simulink model "TSR_Scenario_005_cs"  (R2014b)
settings: Solver=ode5  SolverMode=SingleTasking  StartTime=0.0  StopTime=inf  FixedStep=1/100  RelTol=1e-3
PreLoadFcn:
  | mbxruntime.callbacks.PreLoadFcn(bdroot);
  | check_NUTS_defined;
  | 
  | assignin('base',['model_closed_' bdroot],false);
  | 
  | addpath('../includes_TSR/includes_TSR');
  | 
  | switch version('-release')
  | case {'2010a', '2010b', '2011a'}
  | addpath('../includes_TSR/ML2010b');
  | otherwise
  | addpath('../includes_TSR/ML2011b');
  | end
PostLoadFcn:
  | mbxruntime.callbacks.PostLoadFcn(bdroot);
InitFcn:
  | mbxruntime.callbacks.InitFcn(bdroot);
StartFcn:
  | mbxruntime.callbacks.StartFcn(bdroot);
StopFcn:
  | mbxruntime.callbacks.StopFcn(bdroot);
model workspace: external: MAT-File .\TSR_Scenario_005_cs_hws.mat (data not in the file)
undefined symbols (not defined in the file or in its folder): InitImageOutputDir, mbxruntime, OrientationPitch, OrientationRoll, PositionX, PositionY, PositionZ, tabledata, warningInitialVelocity, x0
undefined symbols (not defined in the file): SteeringColumn, SteeringWheel, TSR_Scenario_005_cs_00431f954bf6ed0a, TSR_Scenario_005_cs_02a6645fe307ce96, TSR_Scenario_005_cs_0e0d17e780cba748, TSR_Scenario_005_cs_0f94700004e304be, TSR_Scenario_005_cs_13e63084604f23c5, TSR_Scenario_005_cs_18da76569b226b1d, TSR_Scenario_005_cs_19a09eb0dceaf389, TSR_Scenario_005_cs_1d6b1ecf339da803, TSR_Scenario_005_cs_219485daa5a5d171, TSR_Scenario_005_cs_221c03cfb0670d1a, TSR_Scenario_005_cs_22611db63f83df91, TSR_Scenario_005_cs_24324341e1f0fdeb, TSR_Scenario_005_cs_248b5be6aaeb4a32, TSR_Scenario_005_cs_26d69342f02903e6, TSR_Scenario_005_cs_28d4639b4eb6a924, TSR_Scenario_005_cs_2a50646ef6121283, TSR_Scenario_005_cs_2addef8764f78195, TSR_Scenario_005_cs_2c78bb6e92f1c73d, TSR_Scenario_005_cs_330b013c7926b8c0, TSR_Scenario_005_cs_33ac55a3a4bfafc5, TSR_Scenario_005_cs_33d6442482a921b6, TSR_Scenario_005_cs_36fcc85960c1dc31, TSR_Scenario_005_cs_38acb22310967a91, TSR_Scenario_005_cs_3e8855054a9c05f5, TSR_Scenario_005_cs_43d01b44652f0f38, TSR_Scenario_005_cs_43d19ecb630bd754, TSR_Scenario_005_cs_4487c76a87b8c5f1, TSR_Scenario_005_cs_44ceee846c318dfb, TSR_Scenario_005_cs_450a3683cbfdd730, TSR_Scenario_005_cs_464618e49e37493a, TSR_Scenario_005_cs_4880b38df4698ab1, TSR_Scenario_005_cs_4a2b3c7d0abca22e, TSR_Scenario_005_cs_4bd204b8239d5406, TSR_Scenario_005_cs_4de8d67ffbf74a19, TSR_Scenario_005_cs_4f6170ee339e194e, TSR_Scenario_005_cs_50430c8166448bfc, TSR_Scenario_005_cs_53c8f6734eaacbd2, TSR_Scenario_005_cs_543db9a2ff458ebe, TSR_Scenario_005_cs_57976f30ab2edad5, TSR_Scenario_005_cs_5922fccf31372278, TSR_Scenario_005_cs_5a258c940bbe826b, TSR_Scenario_005_cs_6087cc283675db35, TSR_Scenario_005_cs_6246b869963d4acb, TSR_Scenario_005_cs_6352b9f9b72630f9, TSR_Scenario_005_cs_6559b64eceddc3ca, TSR_Scenario_005_cs_6832a8ea8fa66aa4, TSR_Scenario_005_cs_696d53dba69844e5, TSR_Scenario_005_cs_6cabbb37c4ac2dd1, TSR_Scenario_005_cs_6d528aa494c8a952, TSR_Scenario_005_cs_6d945b49f7234fd2, TSR_Scenario_005_cs_6e2ebc771acb2455, TSR_Scenario_005_cs_7897f864ad990cf0, TSR_Scenario_005_cs_7978c65fd141f076, TSR_Scenario_005_cs_7a9ba94120bbe2c7, TSR_Scenario_005_cs_7b108592703c2dc5, TSR_Scenario_005_cs_7cd2f5b09394b811, TSR_Scenario_005_cs_7e1904d085d8f37f, TSR_Scenario_005_cs_7e555208507e0618 ... (+95)
libraries: simulink_extras x59, PreScanSimulinkLibrary x43, simulink x29
(part 12 of 24)

== system TSR_Scenario_005_cs/VISUColorRegion_Shoes_Male_Regular_wSuitcase_1 ==
  VISUColorRegion_Shoes_Male_Regular_wSuitcase_1 : Inport  Tag=inport/ColorRegion  OutDataTypeStr=Bus: PRESCAN_COLOR_DATA  PortDimensions=1  SampleTime=1/100  BusOutputAsStruct=on
  Actuator : S-Function  FunctionName=sfun_ColorActuator  Parameters=mbxruntime.parameters.convert(UniqueID), mbxruntime.parameters.convert(WorldModelSubPath),tabledata, TimeStep  EnableBusSupport=off  mask(PreScan Sink Block: VisuTextureColor){UniqueID=548, WorldModelSubPath=/recolorRegion:name=Shoes/targetColor, TimeStep=1/100}
      mask prompts: UniqueID "Parent Unique Identifier (auto-generated)"; WorldModelSubPath "WM SubPath(auto-generated)"; TimeStep "Simulink time step"
      mask help:
      | The VisuTextureColor block provides a way to adapt the color of a vehicle.
      |
      | For more information, please click Help.
      mask init:
      | [tabledata] = mbxruntime.parameters.table(UniqueID,WorldModelSubPath);
      mask Help: eval('openHelp(230)')
      mask Display: image(imread('TextureColor.png'))
  wires:
  VISUColorRegion_Shoes_Male_Regular_wSuitcase_1/1 -> Actuator/1

== system TSR_Scenario_005_cs/VISUColorRegion_Upper_Body_Female_RegularAni_1 ==
  VISUColorRegion_Upper_Body_Female_RegularAni_1 : Inport  Tag=inport/ColorRegion  OutDataTypeStr=Bus: PRESCAN_COLOR_DATA  PortDimensions=1  SampleTime=1/100  BusOutputAsStruct=on
  Actuator : S-Function  FunctionName=sfun_ColorActuator  Parameters=mbxruntime.parameters.convert(UniqueID), mbxruntime.parameters.convert(WorldModelSubPath),tabledata, TimeStep  EnableBusSupport=off  mask(PreScan Sink Block: VisuTextureColor){UniqueID=592, WorldModelSubPath=/recolorRegion:name=Upper Body/targetColor, TimeStep=1/100}
      mask prompts: UniqueID "Parent Unique Identifier (auto-generated)"; WorldModelSubPath "WM SubPath(auto-generated)"; TimeStep "Simulink time step"
      mask help:
      | The VisuTextureColor block provides a way to adapt the color of a vehicle.
      |
      | For more information, please click Help.
      mask init:
      | [tabledata] = mbxruntime.parameters.table(UniqueID,WorldModelSubPath);
      mask Help: eval('openHelp(230)')
      mask Display: image(imread('TextureColor.png'))
  wires:
  VISUColorRegion_Upper_Body_Female_RegularAni_1/1 -> Actuator/1

== system TSR_Scenario_005_cs/VISUColorRegion_Upper_Body_Female_Regular_wBuggy_1 ==
  VISUColorRegion_Upper_Body_Female_Regular_wBuggy_1 : Inport  Tag=inport/ColorRegion  OutDataTypeStr=Bus: PRESCAN_COLOR_DATA  PortDimensions=1  SampleTime=1/100  BusOutputAsStruct=on
  Actuator : S-Function  FunctionName=sfun_ColorActuator  Parameters=mbxruntime.parameters.convert(UniqueID), mbxruntime.parameters.convert(WorldModelSubPath),tabledata, TimeStep  EnableBusSupport=off  mask(PreScan Sink Block: VisuTextureColor){UniqueID=539, WorldModelSubPath=/recolorRegion:name=Upper Body/targetColor, TimeStep=1/100}
      mask prompts: UniqueID "Parent Unique Identifier (auto-generated)"; WorldModelSubPath "WM SubPath(auto-generated)"; TimeStep "Simulink time step"
      mask help:
      | The VisuTextureColor block provides a way to adapt the color of a vehicle.
      |
      | For more information, please click Help.
      mask init:
      | [tabledata] = mbxruntime.parameters.table(UniqueID,WorldModelSubPath);
      mask Help: eval('openHelp(230)')
      mask Display: image(imread('TextureColor.png'))
  wires:
  VISUColorRegion_Upper_Body_Female_Regular_wBuggy_1/1 -> Actuator/1

== system TSR_Scenario_005_cs/VISUColorRegion_Upper_Body_Male_RegularAni_1 ==
  VISUColorRegion_Upper_Body_Male_RegularAni_1 : Inport  Tag=inport/ColorRegion  OutDataTypeStr=Bus: PRESCAN_COLOR_DATA  PortDimensions=1  SampleTime=1/100  BusOutputAsStruct=on
  Actuator : S-Function  FunctionName=sfun_ColorActuator  Parameters=mbxruntime.parameters.convert(UniqueID), mbxruntime.parameters.convert(WorldModelSubPath),tabledata, TimeStep  EnableBusSupport=off  mask(PreScan Sink Block: VisuTextureColor){UniqueID=316, WorldModelSubPath=/recolorRegion:name=Upper Body/targetColor, TimeStep=1/100}
      mask prompts: UniqueID "Parent Unique Identifier (auto-generated)"; WorldModelSubPath "WM SubPath(auto-generated)"; TimeStep "Simulink time step"
      mask help:
      | The VisuTextureColor block provides a way to adapt the color of a vehicle.
      |
      | For more information, please click Help.
      mask init:
      | [tabledata] = mbxruntime.parameters.table(UniqueID,WorldModelSubPath);
      mask Help: eval('openHelp(230)')
      mask Display: image(imread('TextureColor.png'))
  wires:
  VISUColorRegion_Upper_Body_Male_RegularAni_1/1 -> Actuator/1

== system TSR_Scenario_005_cs/VISUColorRegion_Upper_Body_Male_Regular_wBackpack_1 ==
  VISUColorRegion_Upper_Body_Male_Regular_wBackpack_1 : Inport  Tag=inport/ColorRegion  OutDataTypeStr=Bus: PRESCAN_COLOR_DATA  PortDimensions=1  SampleTime=1/100  BusOutputAsStruct=on
  Actuator : S-Function  FunctionName=sfun_ColorActuator  Parameters=mbxruntime.parameters.convert(UniqueID), mbxruntime.parameters.convert(WorldModelSubPath),tabledata, TimeStep  EnableBusSupport=off  mask(PreScan Sink Block: VisuTextureColor){UniqueID=595, WorldModelSubPath=/recolorRegion:name=Upper Body/targetColor, TimeStep=1/100}
      mask prompts: UniqueID "Parent Unique Identifier (auto-generated)"; WorldModelSubPath "WM SubPath(auto-generated)"; TimeStep "Simulink time step"
      mask help:
      | The VisuTextureColor block provides a way to adapt the color of a vehicle.
      |
      | For more information, please click Help.
      mask init:
      | [tabledata] = mbxruntime.parameters.table(UniqueID,WorldModelSubPath);
      mask Help: eval('openHelp(230)')
      mask Display: image(imread('TextureColor.png'))
  wires:
  VISUColorRegion_Upper_Body_Male_Regular_wBackpack_1/1 -> Actuator/1

== system TSR_Scenario_005_cs/VISUColorRegion_Upper_Body_Male_Regular_wBicycle_1 ==
  VISUColorRegion_Upper_Body_Male_Regular_wBicycle_1 : Inport  Tag=inport/ColorRegion  OutDataTypeStr=Bus: PRESCAN_COLOR_DATA  PortDimensions=1  SampleTime=1/100  BusOutputAsStruct=on
  Actuator : S-Function  FunctionName=sfun_ColorActuator  Parameters=mbxruntime.parameters.convert(UniqueID), mbxruntime.parameters.convert(WorldModelSubPath),tabledata, TimeStep  EnableBusSupport=off  mask(PreScan Sink Block: VisuTextureColor){UniqueID=542, WorldModelSubPath=/recolorRegion:name=Upper Body/targetColor, TimeStep=1/100}
      mask prompts: UniqueID "Parent Unique Identifier (auto-generated)"; WorldModelSubPath "WM SubPath(auto-generated)"; TimeStep "Simulink time step"
      mask help:
      | The VisuTextureColor block provides a way to adapt the color of a vehicle.
      |
      | For more information, please click Help.
      mask init:
      | [tabledata] = mbxruntime.parameters.table(UniqueID,WorldModelSubPath);
      mask Help: eval('openHelp(230)')
      mask Display: image(imread('TextureColor.png'))
  wires:
  VISUColorRegion_Upper_Body_Male_Regular_wBicycle_1/1 -> Actuator/1

== system TSR_Scenario_005_cs/VISUColorRegion_Upper_Body_Male_Regular_wSuitcase_1 ==
  VISUColorRegion_Upper_Body_Male_Regular_wSuitcase_1 : Inport  Tag=inport/ColorRegion  OutDataTypeStr=Bus: PRESCAN_COLOR_DATA  PortDimensions=1  SampleTime=1/100  BusOutputAsStruct=on
  Actuator : S-Function  FunctionName=sfun_ColorActuator  Parameters=mbxruntime.parameters.convert(UniqueID), mbxruntime.parameters.convert(WorldModelSubPath),tabledata, TimeStep  EnableBusSupport=off  mask(PreScan Sink Block: VisuTextureColor){UniqueID=548, WorldModelSubPath=/recolorRegion:name=Upper Body/targetColor, TimeStep=1/100}
      mask prompts: UniqueID "Parent Unique Identifier (auto-generated)"; WorldModelSubPath "WM SubPath(auto-generated)"; TimeStep "Simulink time step"
      mask help:
      | The VisuTextureColor block provides a way to adapt the color of a vehicle.
      |
      | For more information, please click Help.
      mask init:
      | [tabledata] = mbxruntime.parameters.table(UniqueID,WorldModelSubPath);
      mask Help: eval('openHelp(230)')
      mask Display: image(imread('TextureColor.png'))
  wires:
  VISUColorRegion_Upper_Body_Male_Regular_wSuitcase_1/1 -> Actuator/1

== system TSR_Scenario_005_cs/WheelL0_Audi_A8_1 ==
  WheelL0_Audi_A8_1 : Inport  Tag=inport/JointActuator  OutDataTypeStr=Bus: PRESCAN_POSE_DATA  SampleTime=1/100  BusOutputAsStruct=on
  Actuator : Subsystem  Tag=VisuJoint  mask(PreScan Sink Block: VisuJoint){UniqueID=210, Translate_ObjectID3D=Audi_A8_1.WheelL0, Rotate_ObjectID3D=Audi_A8_1.WheelL0, TimeStep=1/100, DisplayName=[]}
      mask prompts: UniqueID "Parent Unique ID"; Translate_ObjectID3D "Translate Object Name"; Rotate_ObjectID3D "Rotate Object Name"; TimeStep "Simulation Step"; DisplayName "Display Name"
      mask help:
      | The VisuJoint block provides a way to adapt the location and orientation of a part of an object.
      |
      | For more information, please click Help.
      settings: DeleteFcn=PreScanBlockDeleteFcn;
      mask Help: eval('openHelp(223)')
      mask Display: image(imread('Joint.png'))
  wires:
  WheelL0_Audi_A8_1/1 -> Actuator/1(Joint)

== system TSR_Scenario_005_cs/WheelL0_Ford_Fiesta_1 ==
  WheelL0_Ford_Fiesta_1 : Inport  Tag=inport/JointActuator  OutDataTypeStr=Bus: PRESCAN_POSE_DATA  SampleTime=1/100  BusOutputAsStruct=on
  Actuator : Subsystem  Tag=VisuJoint  mask(PreScan Sink Block: VisuJoint){UniqueID=231, Translate_ObjectID3D=Ford_Fiesta_1.WheelL0, Rotate_ObjectID3D=Ford_Fiesta_1.WheelL0, TimeStep=1/100, DisplayName=[]}
      mask prompts: UniqueID "Parent Unique ID"; Translate_ObjectID3D "Translate Object Name"; Rotate_ObjectID3D "Rotate Object Name"; TimeStep "Simulation Step"; DisplayName "Display Name"
      mask help:
      | The VisuJoint block provides a way to adapt the location and orientation of a part of an object.
      |
      | For more information, please click Help.
      settings: DeleteFcn=PreScanBlockDeleteFcn;
      mask Help: eval('openHelp(223)')
      mask Display: image(imread('Joint.png'))
  wires:
  WheelL0_Ford_Fiesta_1/1 -> Actuator/1(Joint)

== system TSR_Scenario_005_cs/WheelL0_Toyota_Yaris_1 ==
  WheelL0_Toyota_Yaris_1 : Inport  Tag=inport/JointActuator  OutDataTypeStr=Bus: PRESCAN_POSE_DATA  SampleTime=1/100  BusOutputAsStruct=on
  Actuator : Subsystem  Tag=VisuJoint  mask(PreScan Sink Block: VisuJoint){UniqueID=225, Translate_ObjectID3D=Toyota_Yaris_1.WheelL0, Rotate_ObjectID3D=Toyota_Yaris_1.WheelL0, TimeStep=1/100, DisplayName=[]}
      mask prompts: UniqueID "Parent Unique ID"; Translate_ObjectID3D "Translate Object Name"; Rotate_ObjectID3D "Rotate Object Name"; TimeStep "Simulation Step"; DisplayName "Display Name"
      mask help:
      | The VisuJoint block provides a way to adapt the location and orientation of a part of an object.
      |
      | For more information, please click Help.
      settings: DeleteFcn=PreScanBlockDeleteFcn;
      mask Help: eval('openHelp(223)')
      mask Display: image(imread('Joint.png'))
  wires:
  WheelL0_Toyota_Yaris_1/1 -> Actuator/1(Joint)

== system TSR_Scenario_005_cs/WheelL1_Audi_A8_1 ==
  WheelL1_Audi_A8_1 : Inport  Tag=inport/JointActuator  OutDataTypeStr=Bus: PRESCAN_POSE_DATA  SampleTime=1/100  BusOutputAsStruct=on
  Actuator : Subsystem  Tag=VisuJoint  mask(PreScan Sink Block: VisuJoint){UniqueID=210, Translate_ObjectID3D=Audi_A8_1.WheelL1, Rotate_ObjectID3D=Audi_A8_1.WheelL1, TimeStep=1/100, DisplayName=[]}
      mask prompts: UniqueID "Parent Unique ID"; Translate_ObjectID3D "Translate Object Name"; Rotate_ObjectID3D "Rotate Object Name"; TimeStep "Simulation Step"; DisplayName "Display Name"
      mask help:
      | The VisuJoint block provides a way to adapt the location and orientation of a part of an object.
      |
      | For more information, please click Help.
      settings: DeleteFcn=PreScanBlockDeleteFcn;
      mask Help: eval('openHelp(223)')
      mask Display: image(imread('Joint.png'))
  wires:
  WheelL1_Audi_A8_1/1 -> Actuator/1(Joint)

== system TSR_Scenario_005_cs/WheelL1_Ford_Fiesta_1 ==
  WheelL1_Ford_Fiesta_1 : Inport  Tag=inport/JointActuator  OutDataTypeStr=Bus: PRESCAN_POSE_DATA  SampleTime=1/100  BusOutputAsStruct=on
  Actuator : Subsystem  Tag=VisuJoint  mask(PreScan Sink Block: VisuJoint){UniqueID=231, Translate_ObjectID3D=Ford_Fiesta_1.WheelL1, Rotate_ObjectID3D=Ford_Fiesta_1.WheelL1, TimeStep=1/100, DisplayName=[]}
      mask prompts: UniqueID "Parent Unique ID"; Translate_ObjectID3D "Translate Object Name"; Rotate_ObjectID3D "Rotate Object Name"; TimeStep "Simulation Step"; DisplayName "Display Name"
      mask help:
      | The VisuJoint block provides a way to adapt the location and orientation of a part of an object.
      |
      | For more information, please click Help.
      settings: DeleteFcn=PreScanBlockDeleteFcn;
      mask Help: eval('openHelp(223)')
      mask Display: image(imread('Joint.png'))
  wires:
  WheelL1_Ford_Fiesta_1/1 -> Actuator/1(Joint)

== system TSR_Scenario_005_cs/WheelL1_Toyota_Yaris_1 ==
  WheelL1_Toyota_Yaris_1 : Inport  Tag=inport/JointActuator  OutDataTypeStr=Bus: PRESCAN_POSE_DATA  SampleTime=1/100  BusOutputAsStruct=on
  Actuator : Subsystem  Tag=VisuJoint  mask(PreScan Sink Block: VisuJoint){UniqueID=225, Translate_ObjectID3D=Toyota_Yaris_1.WheelL1, Rotate_ObjectID3D=Toyota_Yaris_1.WheelL1, TimeStep=1/100, DisplayName=[]}
      mask prompts: UniqueID "Parent Unique ID"; Translate_ObjectID3D "Translate Object Name"; Rotate_ObjectID3D "Rotate Object Name"; TimeStep "Simulation Step"; DisplayName "Display Name"
      mask help:
      | The VisuJoint block provides a way to adapt the location and orientation of a part of an object.
      |
      | For more information, please click Help.
      settings: DeleteFcn=PreScanBlockDeleteFcn;
      mask Help: eval('openHelp(223)')
      mask Display: image(imread('Joint.png'))
  wires:
  WheelL1_Toyota_Yaris_1/1 -> Actuator/1(Joint)

== system TSR_Scenario_005_cs/WheelR0_Audi_A8_1 ==
  WheelR0_Audi_A8_1 : Inport  Tag=inport/JointActuator  OutDataTypeStr=Bus: PRESCAN_POSE_DATA  SampleTime=1/100  BusOutputAsStruct=on
  Actuator : Subsystem  Tag=VisuJoint  mask(PreScan Sink Block: VisuJoint){UniqueID=210, Translate_ObjectID3D=Audi_A8_1.WheelR0, Rotate_ObjectID3D=Audi_A8_1.WheelR0, TimeStep=1/100, DisplayName=[]}
      mask prompts: UniqueID "Parent Unique ID"; Translate_ObjectID3D "Translate Object Name"; Rotate_ObjectID3D "Rotate Object Name"; TimeStep "Simulation Step"; DisplayName "Display Name"
      mask help:
      | The VisuJoint block provides a way to adapt the location and orientation of a part of an object.
      |
      | For more information, please click Help.
      settings: DeleteFcn=PreScanBlockDeleteFcn;
      mask Help: eval('openHelp(223)')
      mask Display: image(imread('Joint.png'))
  wires:
  WheelR0_Audi_A8_1/1 -> Actuator/1(Joint)

== system TSR_Scenario_005_cs/WheelR0_Ford_Fiesta_1 ==
  WheelR0_Ford_Fiesta_1 : Inport  Tag=inport/JointActuator  OutDataTypeStr=Bus: PRESCAN_POSE_DATA  SampleTime=1/100  BusOutputAsStruct=on
  Actuator : Subsystem  Tag=VisuJoint  mask(PreScan Sink Block: VisuJoint){UniqueID=231, Translate_ObjectID3D=Ford_Fiesta_1.WheelR0, Rotate_ObjectID3D=Ford_Fiesta_1.WheelR0, TimeStep=1/100, DisplayName=[]}
      mask prompts: UniqueID "Parent Unique ID"; Translate_ObjectID3D "Translate Object Name"; Rotate_ObjectID3D "Rotate Object Name"; TimeStep "Simulation Step"; DisplayName "Display Name"
      mask help:
      | The VisuJoint block provides a way to adapt the location and orientation of a part of an object.
      |
      | For more information, please click Help.
      settings: DeleteFcn=PreScanBlockDeleteFcn;
      mask Help: eval('openHelp(223)')
      mask Display: image(imread('Joint.png'))
  wires:
  WheelR0_Ford_Fiesta_1/1 -> Actuator/1(Joint)

== system TSR_Scenario_005_cs/WheelR0_Toyota_Yaris_1 ==
  WheelR0_Toyota_Yaris_1 : Inport  Tag=inport/JointActuator  OutDataTypeStr=Bus: PRESCAN_POSE_DATA  SampleTime=1/100  BusOutputAsStruct=on
  Actuator : Subsystem  Tag=VisuJoint  mask(PreScan Sink Block: VisuJoint){UniqueID=225, Translate_ObjectID3D=Toyota_Yaris_1.WheelR0, Rotate_ObjectID3D=Toyota_Yaris_1.WheelR0, TimeStep=1/100, DisplayName=[]}
      mask prompts: UniqueID "Parent Unique ID"; Translate_ObjectID3D "Translate Object Name"; Rotate_ObjectID3D "Rotate Object Name"; TimeStep "Simulation Step"; DisplayName "Display Name"
      mask help:
      | The VisuJoint block provides a way to adapt the location and orientation of a part of an object.
      |
      | For more information, please click Help.
      settings: DeleteFcn=PreScanBlockDeleteFcn;
      mask Help: eval('openHelp(223)')
      mask Display: image(imread('Joint.png'))
  wires:
  WheelR0_Toyota_Yaris_1/1 -> Actuator/1(Joint)

== system TSR_Scenario_005_cs/WheelR1_Audi_A8_1 ==
  WheelR1_Audi_A8_1 : Inport  Tag=inport/JointActuator  OutDataTypeStr=Bus: PRESCAN_POSE_DATA  SampleTime=1/100  BusOutputAsStruct=on
  Actuator : Subsystem  Tag=VisuJoint  mask(PreScan Sink Block: VisuJoint){UniqueID=210, Translate_ObjectID3D=Audi_A8_1.WheelR1, Rotate_ObjectID3D=Audi_A8_1.WheelR1, TimeStep=1/100, DisplayName=[]}
      mask prompts: UniqueID "Parent Unique ID"; Translate_ObjectID3D "Translate Object Name"; Rotate_ObjectID3D "Rotate Object Name"; TimeStep "Simulation Step"; DisplayName "Display Name"
      mask help:
      | The VisuJoint block provides a way to adapt the location and orientation of a part of an object.
      |
      | For more information, please click Help.
      settings: DeleteFcn=PreScanBlockDeleteFcn;
      mask Help: eval('openHelp(223)')
      mask Display: image(imread('Joint.png'))
  wires:
  WheelR1_Audi_A8_1/1 -> Actuator/1(Joint)

== system TSR_Scenario_005_cs/WheelR1_Ford_Fiesta_1 ==
  WheelR1_Ford_Fiesta_1 : Inport  Tag=inport/JointActuator  OutDataTypeStr=Bus: PRESCAN_POSE_DATA  SampleTime=1/100  BusOutputAsStruct=on
  Actuator : Subsystem  Tag=VisuJoint  mask(PreScan Sink Block: VisuJoint){UniqueID=231, Translate_ObjectID3D=Ford_Fiesta_1.WheelR1, Rotate_ObjectID3D=Ford_Fiesta_1.WheelR1, TimeStep=1/100, DisplayName=[]}
      mask prompts: UniqueID "Parent Unique ID"; Translate_ObjectID3D "Translate Object Name"; Rotate_ObjectID3D "Rotate Object Name"; TimeStep "Simulation Step"; DisplayName "Display Name"
      mask help:
      | The VisuJoint block provides a way to adapt the location and orientation of a part of an object.
      |
      | For more information, please click Help.
      settings: DeleteFcn=PreScanBlockDeleteFcn;
      mask Help: eval('openHelp(223)')
      mask Display: image(imread('Joint.png'))
  wires:
  WheelR1_Ford_Fiesta_1/1 -> Actuator/1(Joint)

== system TSR_Scenario_005_cs/WheelR1_Toyota_Yaris_1 ==
  WheelR1_Toyota_Yaris_1 : Inport  Tag=inport/JointActuator  OutDataTypeStr=Bus: PRESCAN_POSE_DATA  SampleTime=1/100  BusOutputAsStruct=on
  Actuator : Subsystem  Tag=VisuJoint  mask(PreScan Sink Block: VisuJoint){UniqueID=225, Translate_ObjectID3D=Toyota_Yaris_1.WheelR1, Rotate_ObjectID3D=Toyota_Yaris_1.WheelR1, TimeStep=1/100, DisplayName=[]}
      mask prompts: UniqueID "Parent Unique ID"; Translate_ObjectID3D "Translate Object Name"; Rotate_ObjectID3D "Rotate Object Name"; TimeStep "Simulation Step"; DisplayName "Display Name"
      mask help:
      | The VisuJoint block provides a way to adapt the location and orientation of a part of an object.
      |
      | For more information, please click Help.
      settings: DeleteFcn=PreScanBlockDeleteFcn;
      mask Help: eval('openHelp(223)')
      mask Display: image(imread('Joint.png'))
  wires:
  WheelR1_Toyota_Yaris_1/1 -> Actuator/1(Joint)

== system TSR_Scenario_005_cs/Actros_1860_1/SELF_Demux ==
  SELF : Inport  OutDataTypeStr=Bus: PRESCAN_SELFSENSORDATA
  Bus Selector : BusSelector  OutputSignals=PositionX,PositionY,PositionZ,OrientationRoll,OrientationPitch,OrientationYaw,Velocity,Yaw_rate,Lat,Long,Alt
  Demux2 : Demux  Outputs=3
  Gain : Gain  Gain=180/pi
  Gain1 : Gain  Gain=180/pi
  Vector Concatenate1 : Concatenate  NumInputs=3
  compas converter : Subsystem
  x [m] : Outport
  y [m] : Outport  Port=2
  z [m] : Outport  Port=3
  rotx [deg] : Outport  Port=4
  roty [deg] : Outport  Port=5
  rotz [deg] : Outport  Port=6
  GPS lat [deg] : Outport  Port=7
  GPS long [deg] : Outport  Port=8
  GPS alt [m] : Outport  Port=9
  velocity [m/s] : Outport  Port=10
  heading [deg] : Outport  Port=11
  yaw rate [deg/s] : Outport  Port=12
  wires:
  Bus Selector/11 -> GPS alt [m]/1  "<Alt>"
  Bus Selector/10 -> GPS long [deg]/1  "<Long>"
  Bus Selector/9 -> GPS lat [deg]/1  "<Lat>"
  Bus Selector/8 -> Gain1/1  "<Yaw_rate>"
  Bus Selector/7 -> velocity [m/s]/1  "<Velocity>"
  Bus Selector/6 -> compas converter/1(rotz [rad]), Vector Concatenate1/3  "<OrientationYaw>"
  Bus Selector/5 -> Vector Concatenate1/2  "<OrientationPitch>"
  Bus Selector/4 -> Vector Concatenate1/1  "<OrientationRoll>"
  Vector Concatenate1/1 -> Gain/1
  Bus Selector/3 -> z [m]/1  "<PositionZ>"
  Bus Selector/2 -> y [m]/1  "<PositionY>"
  Bus Selector/1 -> x [m]/1  "<PositionX>"
  SELF/1 -> Bus Selector/1
  Gain/1 -> Demux2/1
  Demux2/1 -> rotx [deg]/1
  Demux2/2 -> roty [deg]/1
  Demux2/3 -> rotz [deg]/1
  compas converter/1(heading [deg]) -> heading [deg]/1
  Gain1/1 -> yaw rate [deg/s]/1

== system TSR_Scenario_005_cs/Actros_2541_1/Dynamics_Empty ==
  note: For state mode 'Dynamic' positions
      | are not taken into account, as they
      | are computed by integrating velocity.
      | Click annotation for Help.
  Ground_{1..9} (9 alike) : Ground
  MuxState : Subsystem  Tag=mux/State  mask(Empty Dynamics State Block){positioningmode=on, TimeStep=1/100}
      mask prompts: positioningmode "Positioning Mode"; TimeStep "Auto Assigned: Time Step [s]"
      mask help:
      | Build the state of an actor based on user input.
      | The user can either use positioning mode or dynamics mode.
      | - When using positioning mode the position and orientation of the actor are set directly based on the input. Expected input is relative to the initial position and orientation of the actor. It's also possible to specify the velocity of the actor, though this input isn't used, only passed on.
      | - When using dynamics mode the position input is ignored. Expected input is velocity and orientation. The velocity is relative the current orientation of the actor, while orientation is relative to its initial orientation. The position of the actor is calculated based on the velocity and orientation given.
      settings: DeleteFcn=PreScanBlockDeleteFcn;
  STATE_Actros_2541_1 : Subsystem  Tag=mux/StatePort  Priority=0  LoadFcn=load PrescanStateActuatorData  mask(PreScan Sink Block: State){x0=TSR_Scenario_005_cs_81f8b291f80d3bb5, y0=TSR_Scenario_005_cs_b36b553bfda2753f, z0=TSR_Scenario_005_cs_ceb708ef07534e98, Roll0=TSR_Scenario_005_cs_7e1904d085d8f37f, Pitch0=TSR_Scenario_005_cs_cf6308a405ae1ed0, Yaw0=TSR_Scenario_005_cs_3e8855054a9c05f5, TimeStep=1/100}
      mask prompts: x0 "Ini x-position VEHICLE wrt GLOBAL axis system [m]"; y0 "Ini y-position VEHICLE wrt GLOBAL axis system [m]"; z0 "Ini z-position VEHICLE wrt GLOBAL axis system [m]"; Roll0 "Ini roll-angle BODY wrt VEHICLE axis system [deg]"; Pitch0 "Ini pitch-angle BODY wrt VEHICLE axis system [deg]"; Yaw0 "Ini yaw-angle VEHICLE wrt GLOBAL axis system [deg]"; TimeStep "Auto-Assigned: Upload Period [s]"
      mask help:
      | The Actor State contains a vector signal of size (9x1), containing the following signals:
      |
      | -  Position                  (x,y,z)                                     [m]
      | -  Velocity                  (vx,vy,vz)                               [m/s]
      | -  Angles                    (Roll, Pitch, Yaw)                   [rad]
      |
      | The Actor state is defined in the global axis system.
      | The state is superponed on the Initial position defined in the GUI.
      |
      | For more information, please click Help.
      settings: DeleteFcn=PreScanBlockDeleteFcn;
      mask Help: eval('openHelp(222)')
      mask Display: image(imread('State.png'))
  State : Outport  Tag=outport/StateOutport  SampleTime=1/100
  wires:
  MuxState/1(state) -> STATE_Actros_2541_1/1(State)
  STATE_Actros_2541_1/1(StateBus) -> State/1
  Ground_1/1 -> MuxState/1(x [m])
  Ground_2/1 -> MuxState/2(y [m])
  Ground_3/1 -> MuxState/3(z [m])
  Ground_4/1 -> MuxState/4(dx [m/s])
  Ground_5/1 -> MuxState/5(dy [m/s])
  Ground_6/1 -> MuxState/6(dz [m/s])
  Ground_7/1 -> MuxState/7(R [rad])
  Ground_8/1 -> MuxState/8(P [rad])
  Ground_9/1 -> MuxState/9(Y [rad])

== system TSR_Scenario_005_cs/Actros_2541_1/SELF_Demux ==
  SELF : Inport  OutDataTypeStr=Bus: PRESCAN_SELFSENSORDATA
  Bus Selector : BusSelector  OutputSignals=PositionX,PositionY,PositionZ,OrientationRoll,OrientationPitch,OrientationYaw,Velocity,Yaw_rate,Lat,Long,Alt
  Demux2 : Demux  Outputs=3
  Gain : Gain  Gain=180/pi
  Gain1 : Gain  Gain=180/pi
  Vector Concatenate1 : Concatenate  NumInputs=3
  compas converter : Subsystem
  x [m] : Outport
  y [m] : Outport  Port=2
  z [m] : Outport  Port=3
  rotx [deg] : Outport  Port=4
  roty [deg] : Outport  Port=5
  rotz [deg] : Outport  Port=6
  GPS lat [deg] : Outport  Port=7
  GPS long [deg] : Outport  Port=8
  GPS alt [m] : Outport  Port=9
  velocity [m/s] : Outport  Port=10
  heading [deg] : Outport  Port=11
  yaw rate [deg/s] : Outport  Port=12
  wires:
  Bus Selector/11 -> GPS alt [m]/1  "<Alt>"
  Bus Selector/10 -> GPS long [deg]/1  "<Long>"
  Bus Selector/9 -> GPS lat [deg]/1  "<Lat>"
  Bus Selector/8 -> Gain1/1  "<Yaw_rate>"
  Bus Selector/7 -> velocity [m/s]/1  "<Velocity>"
  Bus Selector/6 -> compas converter/1(rotz [rad]), Vector Concatenate1/3  "<OrientationYaw>"
  Bus Selector/5 -> Vector Concatenate1/2  "<OrientationPitch>"
  Bus Selector/4 -> Vector Concatenate1/1  "<OrientationRoll>"
  Vector Concatenate1/1 -> Gain/1
  Bus Selector/3 -> z [m]/1  "<PositionZ>"
  Bus Selector/2 -> y [m]/1  "<PositionY>"
  Bus Selector/1 -> x [m]/1  "<PositionX>"
  SELF/1 -> Bus Selector/1
  Gain/1 -> Demux2/1
  Demux2/1 -> rotx [deg]/1
  Demux2/2 -> roty [deg]/1
  Demux2/3 -> rotz [deg]/1
  compas converter/1(heading [deg]) -> heading [deg]/1
  Gain1/1 -> yaw rate [deg/s]/1

== system TSR_Scenario_005_cs/Audi_A8_1/  ==
  rotX [deg] : Inport
  rotY [deg] : Inport  Port=2
  Degrees to Radians : simulink_extras/Transformations/Degrees to Radians
  Degrees to Radians1 : simulink_extras/Transformations/Degrees to Radians
  Demux : Demux
  Gain : Gain  Gain=[a a -b -b]
  Gain1 : Gain  Gain=[-TW TW -TW TW]
  Integer Delay : Delay  DelayLength=1
  Integer Delay1 : Delay  DelayLength=1
  Sum : Sum  Inputs=|++
  Trigonometric Function : Trigonometry
  Trigonometric Function1 : Trigonometry
  zDisp FL [m] : Outport
  zDisp FR [m] : Outport  Port=2
  zDisp RL [m] : Outport  Port=3
  zDisp RR [m] : Outport  Port=4
  wires:
  Gain1/1 -> Sum/2
  Sum/1 -> Demux/1
  Gain/1 -> Sum/1
  Integer Delay1/1 -> Degrees to Radians1/1
  rotX [deg]/1 -> Integer Delay1/1
  Degrees to Radians1/1 -> Trigonometric Function1/1
  Trigonometric Function1/1 -> Gain1/1
  Integer Delay/1 -> Degrees to Radians/1
  rotY [deg]/1 -> Integer Delay/1
  Degrees to Radians/1 -> Trigonometric Function/1
  Trigonometric Function/1 -> Gain/1
  Demux/1 -> zDisp FL [m]/1
  Demux/2 -> zDisp FR [m]/1
  Demux/3 -> zDisp RL [m]/1
  Demux/4 -> zDisp RR [m]/1

== system TSR_Scenario_005_cs/Audi_A8_1/Brake_light_left_Mux ==
  MSCD [Cd] : Inport
  Position (xyz) [m] : Inport  Port=2
  Orientation (RPY) [deg] : Inport  Port=3
  Color [-] : Inport  Port=4
  TextureResourceID [-] : Inport  Port=5
  Bus Creator : BusCreator  Inputs='Intensity','Position','Orientation','Color','TextureResourceID'  OutDataTypeStr=Bus: PRESCAN_VISULIGHTACTUATOR_DATA  NonVirtualBus=on
  Bus Creator1 : BusCreator  Inputs=3  OutDataTypeStr=Bus: PRESCAN_RGB_DATA  NonVirtualBus=on
  Bus Creator2 : BusCreator  Inputs=3  OutDataTypeStr=Bus: PRESCAN_RPY_DATA  NonVirtualBus=on
  Bus Creator3 : BusCreator  Inputs=3  OutDataTypeStr=Bus: PRESCAN_XYZ_DATA  NonVirtualBus=on
  Data Type Conversion : DataTypeConversion  OutDataTypeStr=int32  RndMeth=Nearest
  Degrees to Radians : simulink_extras/Transformations/Degrees to Radians
  Demux : Demux  Outputs=3
  Demux1 : Demux  Outputs=3
  Demux2 : Demux  Outputs=3
  Lights : Outport
  wires:
  TextureResourceID [-]/1 -> Data Type Conversion/1  "TextureResourceID"
  MSCD [Cd]/1 -> Bus Creator/1  "Intensity"
  Bus Creator/1 -> Lights/1
  Demux/1 -> Bus Creator1/1  "R"
  Demux/2 -> Bus Creator1/2  "G"
  Demux/3 -> Bus Creator1/3  "B"
  Color [-]/1 -> Demux/1  "Color"
  Bus Creator1/1 -> Bus Creator/4  "Color"
  Demux1/1 -> Bus Creator2/1  "Roll"
  Demux1/2 -> Bus Creator2/2  "Pitch"
  Demux1/3 -> Bus Creator2/3  "Yaw"
  Orientation (RPY) [deg]/1 -> Degrees to Radians/1  "Orientation"
  Bus Creator2/1 -> Bus Creator/3  "Orientation"
  Demux2/1 -> Bus Creator3/1  "X"
  Demux2/2 -> Bus Creator3/2  "Y"
  Demux2/3 -> Bus Creator3/3  "Z"
  Position (xyz) [m]/1 -> Demux2/1  "Position"
  Bus Creator3/1 -> Bus Creator/2  "Position"
  Data Type Conversion/1 -> Bus Creator/5  "TextureResourceID"
  Degrees to Radians/1 -> Demux1/1

== system TSR_Scenario_005_cs/Audi_A8_1/Brake_light_right_Mux ==
  MSCD [Cd] : Inport
  Position (xyz) [m] : Inport  Port=2
  Orientation (RPY) [deg] : Inport  Port=3
  Color [-] : Inport  Port=4
  TextureResourceID [-] : Inport  Port=5
  Bus Creator : BusCreator  Inputs='Intensity','Position','Orientation','Color','TextureResourceID'  OutDataTypeStr=Bus: PRESCAN_VISULIGHTACTUATOR_DATA  NonVirtualBus=on
  Bus Creator1 : BusCreator  Inputs=3  OutDataTypeStr=Bus: PRESCAN_RGB_DATA  NonVirtualBus=on
  Bus Creator2 : BusCreator  Inputs=3  OutDataTypeStr=Bus: PRESCAN_RPY_DATA  NonVirtualBus=on
  Bus Creator3 : BusCreator  Inputs=3  OutDataTypeStr=Bus: PRESCAN_XYZ_DATA  NonVirtualBus=on
  Data Type Conversion : DataTypeConversion  OutDataTypeStr=int32  RndMeth=Nearest
  Degrees to Radians : simulink_extras/Transformations/Degrees to Radians
  Demux : Demux  Outputs=3
  Demux1 : Demux  Outputs=3
  Demux2 : Demux  Outputs=3
  Lights : Outport
  wires:
  TextureResourceID [-]/1 -> Data Type Conversion/1  "TextureResourceID"
  MSCD [Cd]/1 -> Bus Creator/1  "Intensity"
  Bus Creator/1 -> Lights/1
  Demux/1 -> Bus Creator1/1  "R"
  Demux/2 -> Bus Creator1/2  "G"
  Demux/3 -> Bus Creator1/3  "B"
  Color [-]/1 -> Demux/1  "Color"
  Bus Creator1/1 -> Bus Creator/4  "Color"
  Demux1/1 -> Bus Creator2/1  "Roll"
  Demux1/2 -> Bus Creator2/2  "Pitch"
  Demux1/3 -> Bus Creator2/3  "Yaw"
  Orientation (RPY) [deg]/1 -> Degrees to Radians/1  "Orientation"
  Bus Creator2/1 -> Bus Creator/3  "Orientation"
  Demux2/1 -> Bus Creator3/1  "X"
  Demux2/2 -> Bus Creator3/2  "Y"
  Demux2/3 -> Bus Creator3/3  "Z"
  Position (xyz) [m]/1 -> Demux2/1  "Position"
  Bus Creator3/1 -> Bus Creator/2  "Position"
  Data Type Conversion/1 -> Bus Creator/5  "TextureResourceID"
  Degrees to Radians/1 -> Demux1/1

== system TSR_Scenario_005_cs/Audi_A8_1/CameraSensor_1_CM_Demux ==
  In1 : Inport
  Selector : Selector  NumberOfDimensions=2  InputPortWidth=3  IndexOptions=Index vector (dialog),Index vector (dialog)  Indices=-1,1:hres  OutputSizes=1,1
  Selector1 : Selector  NumberOfDimensions=2  InputPortWidth=3  IndexOptions=Index vector (dialog),Index vector (dialog)  Indices=-1,hres+1:hres*2  OutputSizes=1,1
  Selector2 : Selector  NumberOfDimensions=2  InputPortWidth=3  IndexOptions=Index vector (dialog),Index vector (dialog)  Indices=-1,hres*2+1:hres*3  OutputSizes=1,1
  R : Outport
  G : Outport  Port=2
  B : Outport  Port=3
  wires:
  In1/1 -> Selector1/1, Selector/1, Selector2/1
  Selector/1 -> R/1
  Selector1/1 -> G/1
  Selector2/1 -> B/1

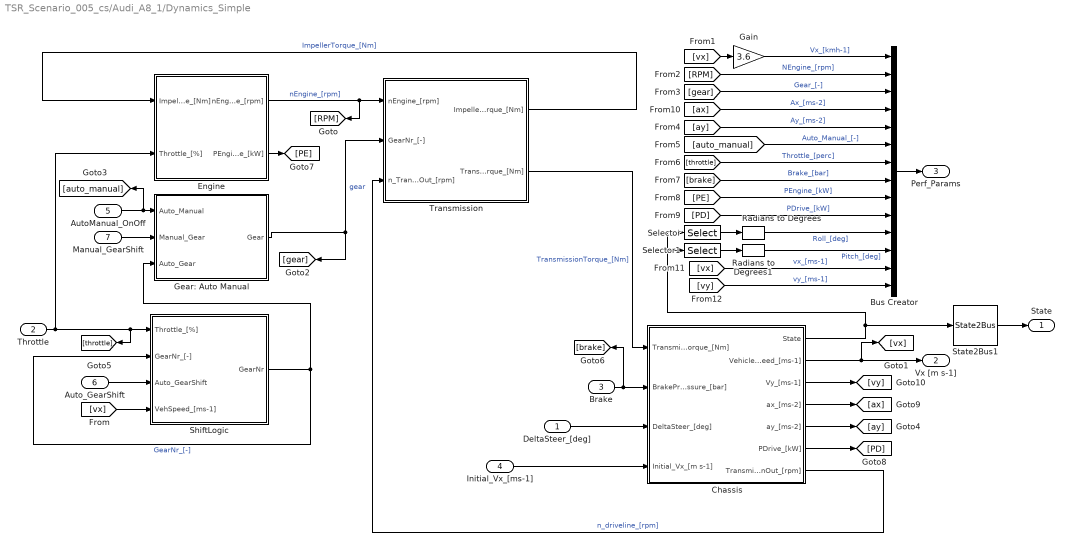
== system TSR_Scenario_005_cs/Audi_A8_1/Dynamics_Simple ==
  DeltaSteer_[deg] : Inport
  Throttle : Inport  Port=2
  Brake : Inport  Port=3
  Initial_Vx_[ms-1] : Inport  Port=4
  AutoManual_OnOff : Inport  Port=5
  Auto_GearShift : Inport  Port=6
  Manual_GearShift : Inport  Port=7
  Bus Creator : BusCreator  Inputs=14
  Chassis : Subsystem
      mask Display: image(imread('Chassis.png'));
  Engine : Subsystem
      mask Display: image(imread('Engine.png'));
  Gain : Gain  Gain=3.6
  Gear: Auto Manual : Subsystem
  Radians to Degrees : simulink_extras/Transformations/Radians to Degrees
  Radians to Degrees1 : simulink_extras/Transformations/Radians to Degrees
  Selector : Selector  InputPortWidth=9  Indices=7
  Selector1 : Selector  InputPortWidth=9  Indices=8
  ShiftLogic : Subsystem
      mask Display: image(imread('Gearshift.png'));
  State2Bus1 : PreScanSimulinkLibrary/State2Bus  Tag=State  Priority=0  x0=initialX  y0=initialY  z0=initialZ  Roll0=initialRoll  Pitch0=initialPitch  Yaw0=initialYaw  TimeStep=TimeStep
  Transmission : Subsystem
      mask Display: image(imread('Transmission.png'));
  State : Outport
  Vx [m s-1] : Outport  Port=2
  Perf_Params : Outport  Port=3
  wires:
  State2Bus1/1 -> State/1
  [vy] -> Bus Creator/14  "vy_[ms-1]"
  [vx] -> Bus Creator/13  "vx_[ms-1]"
  Chassis/7(TransmissionOut_[rpm]) -> Transmission/3(n_TransmissionOut_[rpm])  "n_driveline_[rpm]"
  Chassis/6(PDrive_[kW]) -> [PD]
  Chassis/5(ay_[ms-2]) -> [ay]
  Chassis/4(ax_[ms-2]) -> [ax]
  Chassis/3(Vy_[ms-1]) -> [vy]
  [vx] -> ShiftLogic/4(VehSpeed_[ms-1])
  Gear: Auto Manual/1(Gear) -> Transmission/2(GearNr_[-]), [gear]  "gear"
  Manual_GearShift/1 -> Gear: Auto Manual/2(Manual_Gear)
  AutoManual_OnOff/1 -> Gear: Auto Manual/1(Auto_Manual), [auto_manual]
  Chassis/2(VehicleSpeed_[ms-1]) -> [vx], Vx [m s-1]/1
  Auto_GearShift/1 -> ShiftLogic/3(Auto_GearShift)
  Throttle/1 -> Engine/2(Throttle_[%]), ShiftLogic/1(Throttle_[%]), [throttle]
  Initial_Vx_[ms-1]/1 -> Chassis/4(Initial_Vx_[m s-1])
  DeltaSteer_[deg]/1 -> Chassis/3(DeltaSteer_[deg])
  Chassis/1(State) -> Selector/1, Selector1/1, State2Bus1/1
  Brake/1 -> [brake], Chassis/2(BrakePressure_[bar])
  Engine/1(nEngine_[rpm]) -> [RPM], Transmission/1(nEngine_[rpm])  "nEngine_[rpm]"
  ShiftLogic/1(GearNr) -> Gear: Auto Manual/3(Auto_Gear), ShiftLogic/2(GearNr_[-])  "GearNr_[-]"
  Transmission/2(TransmissionTorque_[Nm]) -> Chassis/1(TransmissionTorque_[Nm])  "TransmissionTorque_[Nm]"
  Transmission/1(ImpellerTorque_[Nm]) -> Engine/1(ImpellerTorque_[Nm])  "ImpellerTorque_[Nm]"
  Gain/1 -> Bus Creator/1  "Vx_[kmh-1]"
  [RPM] -> Bus Creator/2  "NEngine_[rpm]"
  [gear] -> Bus Creator/3  "Gear_[-]"
  [ay] -> Bus Creator/5  "Ay_[ms-2]"
  [auto_manual] -> Bus Creator/6  "Auto_Manual_[-]"
  [throttle] -> Bus Creator/7  "Throttle_[perc]"
  [brake] -> Bus Creator/8  "Brake_[bar]"
  Engine/2(PEngine_[kW]) -> [PE]
  Bus Creator/1 -> Perf_Params/1
  [PE] -> Bus Creator/9  "PEngine_[kW]"
  Radians to Degrees/1 -> Bus Creator/11  "Roll_[deg]"
  Radians to Degrees1/1 -> Bus Creator/12  "Pitch_[deg]"
  [PD] -> Bus Creator/10  "PDrive_[kW]"
  Selector/1 -> Radians to Degrees/1
  Selector1/1 -> Radians to Degrees1/1
  [vx] -> Gain/1
  [ax] -> Bus Creator/4  "Ax_[ms-2]"

== system TSR_Scenario_005_cs/Audi_A8_1/Headlight_HB_left_Mux ==
  MSCD [Cd] : Inport
  Position (xyz) [m] : Inport  Port=2
  Orientation (RPY) [deg] : Inport  Port=3
  Color [-] : Inport  Port=4
  TextureResourceID [-] : Inport  Port=5
  Bus Creator : BusCreator  Inputs='Intensity','Position','Orientation','Color','TextureResourceID'  OutDataTypeStr=Bus: PRESCAN_VISULIGHTACTUATOR_DATA  NonVirtualBus=on
  Bus Creator1 : BusCreator  Inputs=3  OutDataTypeStr=Bus: PRESCAN_RGB_DATA  NonVirtualBus=on
  Bus Creator2 : BusCreator  Inputs=3  OutDataTypeStr=Bus: PRESCAN_RPY_DATA  NonVirtualBus=on
  Bus Creator3 : BusCreator  Inputs=3  OutDataTypeStr=Bus: PRESCAN_XYZ_DATA  NonVirtualBus=on
  Data Type Conversion : DataTypeConversion  OutDataTypeStr=int32  RndMeth=Nearest
  Degrees to Radians : simulink_extras/Transformations/Degrees to Radians
  Demux : Demux  Outputs=3
  Demux1 : Demux  Outputs=3
  Demux2 : Demux  Outputs=3
  Lights : Outport
  wires:
  TextureResourceID [-]/1 -> Data Type Conversion/1  "TextureResourceID"
  MSCD [Cd]/1 -> Bus Creator/1  "Intensity"
  Bus Creator/1 -> Lights/1
  Demux/1 -> Bus Creator1/1  "R"
  Demux/2 -> Bus Creator1/2  "G"
  Demux/3 -> Bus Creator1/3  "B"
  Color [-]/1 -> Demux/1  "Color"
  Bus Creator1/1 -> Bus Creator/4  "Color"
  Demux1/1 -> Bus Creator2/1  "Roll"
  Demux1/2 -> Bus Creator2/2  "Pitch"
  Demux1/3 -> Bus Creator2/3  "Yaw"
  Orientation (RPY) [deg]/1 -> Degrees to Radians/1  "Orientation"
  Bus Creator2/1 -> Bus Creator/3  "Orientation"
  Demux2/1 -> Bus Creator3/1  "X"
  Demux2/2 -> Bus Creator3/2  "Y"
  Demux2/3 -> Bus Creator3/3  "Z"
  Position (xyz) [m]/1 -> Demux2/1  "Position"
  Bus Creator3/1 -> Bus Creator/2  "Position"
  Data Type Conversion/1 -> Bus Creator/5  "TextureResourceID"
  Degrees to Radians/1 -> Demux1/1

== system TSR_Scenario_005_cs/Audi_A8_1/Headlight_HB_right_Mux ==
  MSCD [Cd] : Inport
  Position (xyz) [m] : Inport  Port=2
  Orientation (RPY) [deg] : Inport  Port=3
  Color [-] : Inport  Port=4
  TextureResourceID [-] : Inport  Port=5
  Bus Creator : BusCreator  Inputs='Intensity','Position','Orientation','Color','TextureResourceID'  OutDataTypeStr=Bus: PRESCAN_VISULIGHTACTUATOR_DATA  NonVirtualBus=on
  Bus Creator1 : BusCreator  Inputs=3  OutDataTypeStr=Bus: PRESCAN_RGB_DATA  NonVirtualBus=on
  Bus Creator2 : BusCreator  Inputs=3  OutDataTypeStr=Bus: PRESCAN_RPY_DATA  NonVirtualBus=on
  Bus Creator3 : BusCreator  Inputs=3  OutDataTypeStr=Bus: PRESCAN_XYZ_DATA  NonVirtualBus=on
  Data Type Conversion : DataTypeConversion  OutDataTypeStr=int32  RndMeth=Nearest
  Degrees to Radians : simulink_extras/Transformations/Degrees to Radians
  Demux : Demux  Outputs=3
  Demux1 : Demux  Outputs=3
  Demux2 : Demux  Outputs=3
  Lights : Outport
  wires:
  TextureResourceID [-]/1 -> Data Type Conversion/1  "TextureResourceID"
  MSCD [Cd]/1 -> Bus Creator/1  "Intensity"
  Bus Creator/1 -> Lights/1
  Demux/1 -> Bus Creator1/1  "R"
  Demux/2 -> Bus Creator1/2  "G"
  Demux/3 -> Bus Creator1/3  "B"
  Color [-]/1 -> Demux/1  "Color"
  Bus Creator1/1 -> Bus Creator/4  "Color"
  Demux1/1 -> Bus Creator2/1  "Roll"
  Demux1/2 -> Bus Creator2/2  "Pitch"
  Demux1/3 -> Bus Creator2/3  "Yaw"
  Orientation (RPY) [deg]/1 -> Degrees to Radians/1  "Orientation"
  Bus Creator2/1 -> Bus Creator/3  "Orientation"
  Demux2/1 -> Bus Creator3/1  "X"
  Demux2/2 -> Bus Creator3/2  "Y"
  Demux2/3 -> Bus Creator3/3  "Z"
  Position (xyz) [m]/1 -> Demux2/1  "Position"
  Bus Creator3/1 -> Bus Creator/2  "Position"
  Data Type Conversion/1 -> Bus Creator/5  "TextureResourceID"
  Degrees to Radians/1 -> Demux1/1

== system TSR_Scenario_005_cs/Audi_A8_1/Headlight_LB_left_Mux ==
  MSCD [Cd] : Inport
  Position (xyz) [m] : Inport  Port=2
  Orientation (RPY) [deg] : Inport  Port=3
  Color [-] : Inport  Port=4
  TextureResourceID [-] : Inport  Port=5
  Bus Creator : BusCreator  Inputs='Intensity','Position','Orientation','Color','TextureResourceID'  OutDataTypeStr=Bus: PRESCAN_VISULIGHTACTUATOR_DATA  NonVirtualBus=on
  Bus Creator1 : BusCreator  Inputs=3  OutDataTypeStr=Bus: PRESCAN_RGB_DATA  NonVirtualBus=on
  Bus Creator2 : BusCreator  Inputs=3  OutDataTypeStr=Bus: PRESCAN_RPY_DATA  NonVirtualBus=on
  Bus Creator3 : BusCreator  Inputs=3  OutDataTypeStr=Bus: PRESCAN_XYZ_DATA  NonVirtualBus=on
  Data Type Conversion : DataTypeConversion  OutDataTypeStr=int32  RndMeth=Nearest
  Degrees to Radians : simulink_extras/Transformations/Degrees to Radians
  Demux : Demux  Outputs=3
  Demux1 : Demux  Outputs=3
  Demux2 : Demux  Outputs=3
  Lights : Outport
  wires:
  TextureResourceID [-]/1 -> Data Type Conversion/1  "TextureResourceID"
  MSCD [Cd]/1 -> Bus Creator/1  "Intensity"
  Bus Creator/1 -> Lights/1
  Demux/1 -> Bus Creator1/1  "R"
  Demux/2 -> Bus Creator1/2  "G"
  Demux/3 -> Bus Creator1/3  "B"
  Color [-]/1 -> Demux/1  "Color"
  Bus Creator1/1 -> Bus Creator/4  "Color"
  Demux1/1 -> Bus Creator2/1  "Roll"
  Demux1/2 -> Bus Creator2/2  "Pitch"
  Demux1/3 -> Bus Creator2/3  "Yaw"
  Orientation (RPY) [deg]/1 -> Degrees to Radians/1  "Orientation"
  Bus Creator2/1 -> Bus Creator/3  "Orientation"
  Demux2/1 -> Bus Creator3/1  "X"
  Demux2/2 -> Bus Creator3/2  "Y"
  Demux2/3 -> Bus Creator3/3  "Z"
  Position (xyz) [m]/1 -> Demux2/1  "Position"
  Bus Creator3/1 -> Bus Creator/2  "Position"
  Data Type Conversion/1 -> Bus Creator/5  "TextureResourceID"
  Degrees to Radians/1 -> Demux1/1

== system TSR_Scenario_005_cs/Audi_A8_1/Headlight_LB_right_Mux ==
  MSCD [Cd] : Inport
  Position (xyz) [m] : Inport  Port=2
  Orientation (RPY) [deg] : Inport  Port=3
  Color [-] : Inport  Port=4
  TextureResourceID [-] : Inport  Port=5
  Bus Creator : BusCreator  Inputs='Intensity','Position','Orientation','Color','TextureResourceID'  OutDataTypeStr=Bus: PRESCAN_VISULIGHTACTUATOR_DATA  NonVirtualBus=on
  Bus Creator1 : BusCreator  Inputs=3  OutDataTypeStr=Bus: PRESCAN_RGB_DATA  NonVirtualBus=on
  Bus Creator2 : BusCreator  Inputs=3  OutDataTypeStr=Bus: PRESCAN_RPY_DATA  NonVirtualBus=on
  Bus Creator3 : BusCreator  Inputs=3  OutDataTypeStr=Bus: PRESCAN_XYZ_DATA  NonVirtualBus=on
  Data Type Conversion : DataTypeConversion  OutDataTypeStr=int32  RndMeth=Nearest
  Degrees to Radians : simulink_extras/Transformations/Degrees to Radians
  Demux : Demux  Outputs=3
  Demux1 : Demux  Outputs=3
  Demux2 : Demux  Outputs=3
  Lights : Outport
  wires:
  TextureResourceID [-]/1 -> Data Type Conversion/1  "TextureResourceID"
  MSCD [Cd]/1 -> Bus Creator/1  "Intensity"
  Bus Creator/1 -> Lights/1
  Demux/1 -> Bus Creator1/1  "R"
  Demux/2 -> Bus Creator1/2  "G"
  Demux/3 -> Bus Creator1/3  "B"
  Color [-]/1 -> Demux/1  "Color"
  Bus Creator1/1 -> Bus Creator/4  "Color"
  Demux1/1 -> Bus Creator2/1  "Roll"
  Demux1/2 -> Bus Creator2/2  "Pitch"
  Demux1/3 -> Bus Creator2/3  "Yaw"
  Orientation (RPY) [deg]/1 -> Degrees to Radians/1  "Orientation"
  Bus Creator2/1 -> Bus Creator/3  "Orientation"
  Demux2/1 -> Bus Creator3/1  "X"
  Demux2/2 -> Bus Creator3/2  "Y"
  Demux2/3 -> Bus Creator3/3  "Z"
  Position (xyz) [m]/1 -> Demux2/1  "Position"
  Bus Creator3/1 -> Bus Creator/2  "Position"
  Data Type Conversion/1 -> Bus Creator/5  "TextureResourceID"
  Degrees to Radians/1 -> Demux1/1

== system TSR_Scenario_005_cs/Audi_A8_1/Indicator_front_left_Mux ==
  MSCD [Cd] : Inport
  Position (xyz) [m] : Inport  Port=2
  Orientation (RPY) [deg] : Inport  Port=3
  Color [-] : Inport  Port=4
  TextureResourceID [-] : Inport  Port=5
  Bus Creator : BusCreator  Inputs='Intensity','Position','Orientation','Color','TextureResourceID'  OutDataTypeStr=Bus: PRESCAN_VISULIGHTACTUATOR_DATA  NonVirtualBus=on
  Bus Creator1 : BusCreator  Inputs=3  OutDataTypeStr=Bus: PRESCAN_RGB_DATA  NonVirtualBus=on
  Bus Creator2 : BusCreator  Inputs=3  OutDataTypeStr=Bus: PRESCAN_RPY_DATA  NonVirtualBus=on
  Bus Creator3 : BusCreator  Inputs=3  OutDataTypeStr=Bus: PRESCAN_XYZ_DATA  NonVirtualBus=on
  Data Type Conversion : DataTypeConversion  OutDataTypeStr=int32  RndMeth=Nearest
  Degrees to Radians : simulink_extras/Transformations/Degrees to Radians
  Demux : Demux  Outputs=3
  Demux1 : Demux  Outputs=3
  Demux2 : Demux  Outputs=3
  Lights : Outport
  wires:
  TextureResourceID [-]/1 -> Data Type Conversion/1  "TextureResourceID"
  MSCD [Cd]/1 -> Bus Creator/1  "Intensity"
  Bus Creator/1 -> Lights/1
  Demux/1 -> Bus Creator1/1  "R"
  Demux/2 -> Bus Creator1/2  "G"
  Demux/3 -> Bus Creator1/3  "B"
  Color [-]/1 -> Demux/1  "Color"
  Bus Creator1/1 -> Bus Creator/4  "Color"
  Demux1/1 -> Bus Creator2/1  "Roll"
  Demux1/2 -> Bus Creator2/2  "Pitch"
  Demux1/3 -> Bus Creator2/3  "Yaw"
  Orientation (RPY) [deg]/1 -> Degrees to Radians/1  "Orientation"
  Bus Creator2/1 -> Bus Creator/3  "Orientation"
  Demux2/1 -> Bus Creator3/1  "X"
  Demux2/2 -> Bus Creator3/2  "Y"
  Demux2/3 -> Bus Creator3/3  "Z"
  Position (xyz) [m]/1 -> Demux2/1  "Position"
  Bus Creator3/1 -> Bus Creator/2  "Position"
  Data Type Conversion/1 -> Bus Creator/5  "TextureResourceID"
  Degrees to Radians/1 -> Demux1/1

== system TSR_Scenario_005_cs/Audi_A8_1/Indicator_front_right_Mux ==
  MSCD [Cd] : Inport
  Position (xyz) [m] : Inport  Port=2
  Orientation (RPY) [deg] : Inport  Port=3
  Color [-] : Inport  Port=4
  TextureResourceID [-] : Inport  Port=5
  Bus Creator : BusCreator  Inputs='Intensity','Position','Orientation','Color','TextureResourceID'  OutDataTypeStr=Bus: PRESCAN_VISULIGHTACTUATOR_DATA  NonVirtualBus=on
  Bus Creator1 : BusCreator  Inputs=3  OutDataTypeStr=Bus: PRESCAN_RGB_DATA  NonVirtualBus=on
  Bus Creator2 : BusCreator  Inputs=3  OutDataTypeStr=Bus: PRESCAN_RPY_DATA  NonVirtualBus=on
  Bus Creator3 : BusCreator  Inputs=3  OutDataTypeStr=Bus: PRESCAN_XYZ_DATA  NonVirtualBus=on
  Data Type Conversion : DataTypeConversion  OutDataTypeStr=int32  RndMeth=Nearest
  Degrees to Radians : simulink_extras/Transformations/Degrees to Radians
  Demux : Demux  Outputs=3
  Demux1 : Demux  Outputs=3
  Demux2 : Demux  Outputs=3
  Lights : Outport
  wires:
  TextureResourceID [-]/1 -> Data Type Conversion/1  "TextureResourceID"
  MSCD [Cd]/1 -> Bus Creator/1  "Intensity"
  Bus Creator/1 -> Lights/1
  Demux/1 -> Bus Creator1/1  "R"
  Demux/2 -> Bus Creator1/2  "G"
  Demux/3 -> Bus Creator1/3  "B"
  Color [-]/1 -> Demux/1  "Color"
  Bus Creator1/1 -> Bus Creator/4  "Color"
  Demux1/1 -> Bus Creator2/1  "Roll"
  Demux1/2 -> Bus Creator2/2  "Pitch"
  Demux1/3 -> Bus Creator2/3  "Yaw"
  Orientation (RPY) [deg]/1 -> Degrees to Radians/1  "Orientation"
  Bus Creator2/1 -> Bus Creator/3  "Orientation"
  Demux2/1 -> Bus Creator3/1  "X"
  Demux2/2 -> Bus Creator3/2  "Y"
  Demux2/3 -> Bus Creator3/3  "Z"
  Position (xyz) [m]/1 -> Demux2/1  "Position"
  Bus Creator3/1 -> Bus Creator/2  "Position"
  Data Type Conversion/1 -> Bus Creator/5  "TextureResourceID"
  Degrees to Radians/1 -> Demux1/1

== system TSR_Scenario_005_cs/Audi_A8_1/Indicator_rear_left_Mux ==
  MSCD [Cd] : Inport
  Position (xyz) [m] : Inport  Port=2
  Orientation (RPY) [deg] : Inport  Port=3
  Color [-] : Inport  Port=4
  TextureResourceID [-] : Inport  Port=5
  Bus Creator : BusCreator  Inputs='Intensity','Position','Orientation','Color','TextureResourceID'  OutDataTypeStr=Bus: PRESCAN_VISULIGHTACTUATOR_DATA  NonVirtualBus=on
  Bus Creator1 : BusCreator  Inputs=3  OutDataTypeStr=Bus: PRESCAN_RGB_DATA  NonVirtualBus=on
  Bus Creator2 : BusCreator  Inputs=3  OutDataTypeStr=Bus: PRESCAN_RPY_DATA  NonVirtualBus=on
  Bus Creator3 : BusCreator  Inputs=3  OutDataTypeStr=Bus: PRESCAN_XYZ_DATA  NonVirtualBus=on
  Data Type Conversion : DataTypeConversion  OutDataTypeStr=int32  RndMeth=Nearest
  Degrees to Radians : simulink_extras/Transformations/Degrees to Radians
  Demux : Demux  Outputs=3
  Demux1 : Demux  Outputs=3
  Demux2 : Demux  Outputs=3
  Lights : Outport
  wires:
  TextureResourceID [-]/1 -> Data Type Conversion/1  "TextureResourceID"
  MSCD [Cd]/1 -> Bus Creator/1  "Intensity"
  Bus Creator/1 -> Lights/1
  Demux/1 -> Bus Creator1/1  "R"
  Demux/2 -> Bus Creator1/2  "G"
  Demux/3 -> Bus Creator1/3  "B"
  Color [-]/1 -> Demux/1  "Color"
  Bus Creator1/1 -> Bus Creator/4  "Color"
  Demux1/1 -> Bus Creator2/1  "Roll"
  Demux1/2 -> Bus Creator2/2  "Pitch"
  Demux1/3 -> Bus Creator2/3  "Yaw"
  Orientation (RPY) [deg]/1 -> Degrees to Radians/1  "Orientation"
  Bus Creator2/1 -> Bus Creator/3  "Orientation"
  Demux2/1 -> Bus Creator3/1  "X"
  Demux2/2 -> Bus Creator3/2  "Y"
  Demux2/3 -> Bus Creator3/3  "Z"
  Position (xyz) [m]/1 -> Demux2/1  "Position"
  Bus Creator3/1 -> Bus Creator/2  "Position"
  Data Type Conversion/1 -> Bus Creator/5  "TextureResourceID"
  Degrees to Radians/1 -> Demux1/1
